simulink model "sid10"  (R2013a)
settings: Solver=ode45  StartTime=0.0  StopTime=10.0  RelTol=1e-3
libraries: powerlib x6
settings Model: Creator=sidharthbatchu  LastModifiedBy=sidharthbatchu

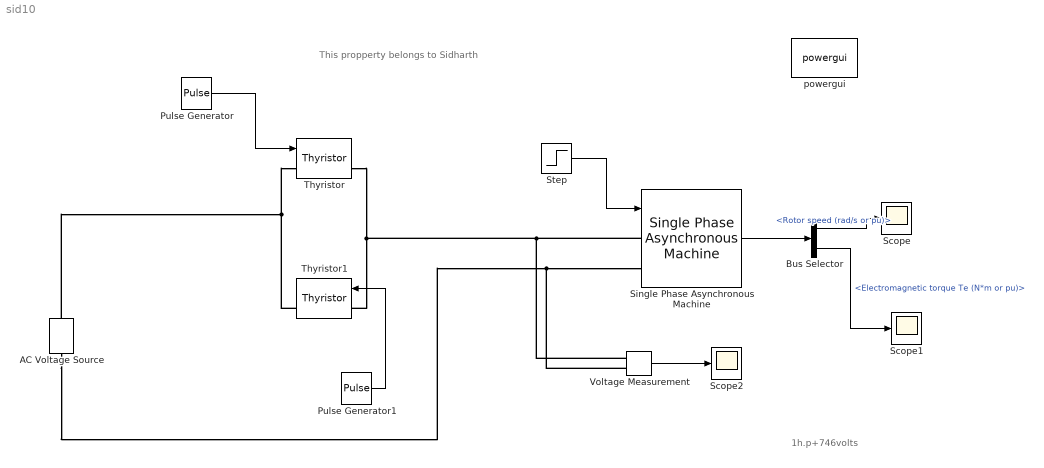
== system sid10 ==
  note: 1h.p+746volts
  note: This propperty belongs to Sidharth
  AC Voltage Source : powerlib/Electrical Sources/AC Voltage Source  Amplitude=100  Phase=0  Frequency=50  SampleTime=0  Measurements=None
  Bus Selector : BusSelector  OutputSignals=Mechanical.Rotor speed (rad/s or pu),Mechanical.Electromagnetic torque Te (N*m or pu)
  Pulse Generator : DiscretePulseGenerator  PulseType=Time based  Amplitude=10  Period=10  PulseWidth=5  PhaseDelay=0.02*(60/360)
  Pulse Generator1 : DiscretePulseGenerator  PulseType=Time based  Period=10  PulseWidth=5  PhaseDelay=0.02*(240/360)
  Scope : Scope
  Scope1 : Scope
  Scope2 : Scope
      settings: SaveName=ScopeData2
  Single Phase Asynchronous Machine : powerlib/Machines/Single Phase Asynchronous Machine  MechanicalLoad=Torque Tm  UNITS=SI  MachineType=Split Phase  NominalParameters="[ .25*746  110  50]"  MainWindingStator="[2.02  7.4e-3]"  MainWindingRotor="[4.12  5.6e-3]"  MutualInductance=0.1772  AuxiliaryWinding="[7.14  8.5e-3]"  Mechanical="[0.0146  0  2 1.18]"  CapacitorStart="[2  254.7e-6]"  CapacitorRun="[18  21.1e-6]"  DisconnectionSpeed=75  InitialSpeed=0  DataType=SI  TsPowergui=0  TsBlock=-1
  Step : Step  SampleTime=0
  Thyristor : powerlib/Power Electronics/Thyristor  Ron=0.001  Lon=0  Vf=0.8  IC=0  Rs=500  Cs=250e-9  Measurements=on
  Thyristor1 : powerlib/Power Electronics/Thyristor  Ron=0.001  Lon=0  Vf=0.8  IC=0  Rs=500  Cs=250e-9  Measurements=on
  Voltage Measurement : powerlib/Measurements/Voltage Measurement  PhasorSimulation=off  OutputType=Complex  PSBequivalent=0
  powergui : powerlib/powergui  Priority=1  SimulationMode=Continuous  SolverType=Tustin  SampleTime=50e-6  frequency=60  SPID=off  DisableSnubberDevices=off  DisableRonSwitches=off  DisableVfSwitches=off  SwTol=0  Interpol=off  DisplayEquations=off  frequencyindice=50  Pbase=100e6  ErrMax=1e-4  Iterations=50  UnitsV=kV  UnitsW=MW  FunctionMessages=off  echomessages=off  HookPort=off  EnableUseOfTLC=off  x0status=blocks  RestoreLinks=warning  ResistiveCurrentMeasurement=off  Frange=[0:2:500]  Ylog=off  Xlog=on  ShowGrid=off  save=off  variable=ZData  ZoomFFT=off  StartTime=0.0  cycles=1  DisplayStyle=1  fundamental=60  FreqAxis=off  MaxFrequency=1000  frequencyindicesteady=1  RmsSteady=1  display=off  Ts=0  methode=off
  wires:
  Bus Selector/1 -> Scope/1  "<Rotor speed (rad/s or pu)>"
  Bus Selector/2 -> Scope1/1  "<Electromagnetic torque Te (N*m or pu)>"
  Single Phase Asynchronous Machine/1 -> Bus Selector/1
  Step/1 -> Single Phase Asynchronous Machine/1
  Pulse Generator/1 -> Thyristor/1
  Pulse Generator1/1 -> Thyristor1/1
  Voltage Measurement/1 -> Scope2/1
  connections:
  Thyristor/RConn1 -- Voltage Measurement/LConn1 -- Single Phase Asynchronous Machine/LConn1 -- Thyristor1/LConn1
  Thyristor1/RConn1 -- AC Voltage Source/RConn1 -- Thyristor/LConn1
  AC Voltage Source/LConn1 -- Voltage Measurement/LConn2 -- Single Phase Asynchronous Machine/LConn2
